simulink model "lab6_model_12b"  (R2012b)
settings: Solver=ode45  StartTime=0.0  StopTime=20  RelTol=1e-3
values from neighbouring files (symbols this model uses):
  A1 = [0 1 0;0 0 1;-11 -6 -13]    [lab6.m]
  A2 = [0 1 0 0; 0 0 1 0; 0 0 0 1; -13 -12 -10 -6]    [lab6.m]
  B1 = [0;0;3]    [lab6.m]
  B2 = [0;0;0;1]    [lab6.m]
  C1 = [1 0 0]    [lab6.m]
  C2 = [2 12 0 0]    [lab6.m]
  D1 = 0    [lab6.m]
  D2 = 0    [lab6.m]
settings Model: Creator=Jessica  LastModifiedBy=Jessica
settings OptimizationCC: ExpressionDepthLimit=128
settings DebuggingCC: UnderspecifiedInitializationDetection=Simplified  MergeDetectMultiDrivingBlocksExec=error  SolverPrmCheckMsg=none  FrameProcessingCompatibilityMsg=error  StateNameClashWarn=none
settings CodeAppCC: CustomSymbolStrType=$N$R$M_T
settings GRTTargetCC: CodeReplacementLibrary=C89/C90 (ANSI)

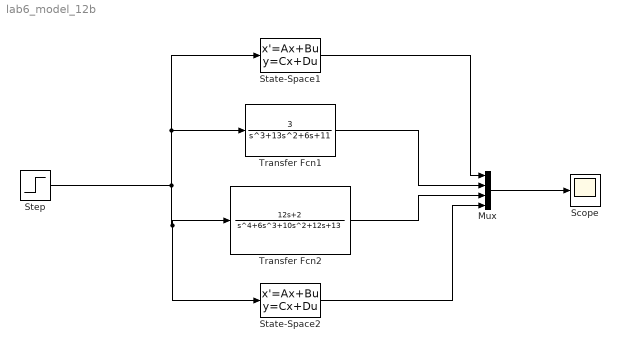
== system lab6_model_12b ==
  Mux : Mux
  Scope : Scope
      settings: SaveName=y
  State-Space1 : StateSpace  A=A1  B=B1  C=C1  D=D1  X0=0
  State-Space2 : StateSpace  A=A2  B=B2  C=C2  D=D2  X0=0
  Step : Step  SampleTime=0
  Transfer Fcn1 : TransferFcn  Numerator=[3]  Denominator=[1 13 6 11]
  Transfer Fcn2 : TransferFcn  Numerator=[12 2]  Denominator=[1 6 10 12 13]
  wires:
  Step/1 -> State-Space2/1, Transfer Fcn2/1, State-Space1/1, Transfer Fcn1/1
  State-Space1/1 -> Mux/1
  Transfer Fcn1/1 -> Mux/2
  Mux/1 -> Scope/1
  Transfer Fcn2/1 -> Mux/3
  State-Space2/1 -> Mux/4
